simulink model "Redresseur_MLI_3Ph_MLI_antiwindup_relay"  (R2018b)
settings: Solver=ode8  StartTime=0.0  StopTime=0.3  FixedStep=1e-6  MaxStep=1e-6  RelTol=1e-3
undefined symbols (not defined in the file): C, Im, inverter_matrix, K, L, R, Ta, Td, Ti, V
libraries: simulink x1
settings Model: Creator=driss  LastModifiedBy=driss
settings SolverCC: ZeroCrossAlgorithm=Adaptive
settings DataIOCC: ReturnWorkspaceOutputs=on
settings DebuggingCC: MaxConsecutiveZCsMsg=none  UnconnectedInputMsg=none  UnconnectedOutputMsg=none  UnconnectedLineMsg=none
settings ModelReferenceCC: EnableRefExpFcnMdlSchedulingChecks=off
settings RTWCC: Description=Generic Real-Time Target

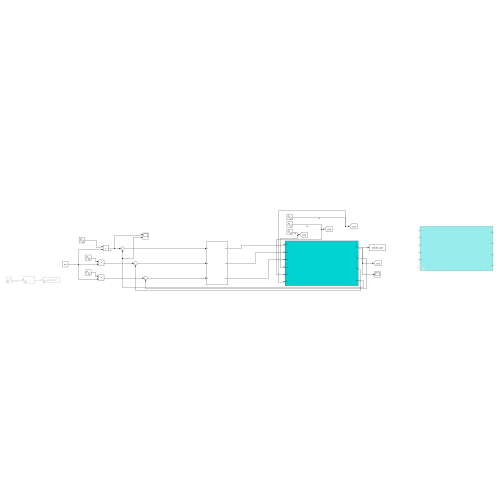
[thumbnail: Simulink's stored preview of the top-level diagram]
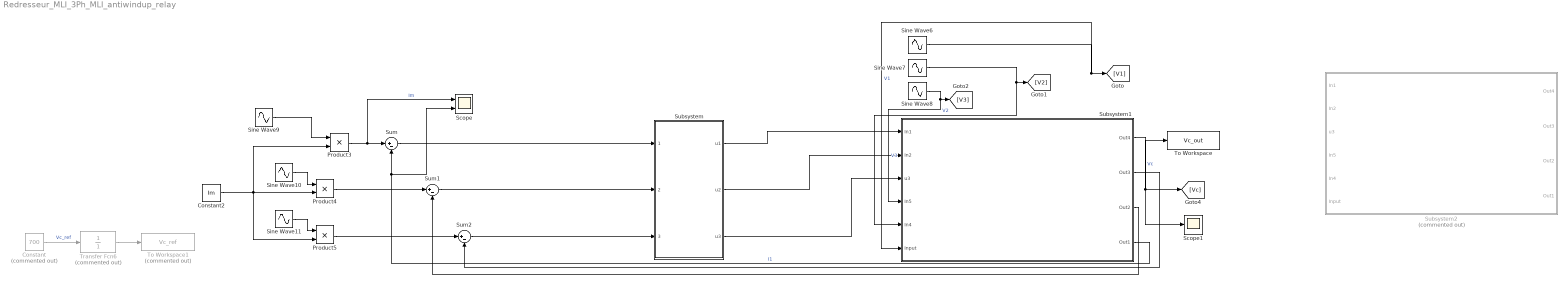
== system Redresseur_MLI_3Ph_MLI_antiwindup_relay ==
  Constant : Constant  Commented=on  Value=700
  Constant2 : Constant  Value=Im
  Product3 : Product
  Product4 : Product
  Product5 : Product
  Scope : Scope  NumInputPorts=2
  Scope1 : Scope
  Sine Wave10 : Sin  Frequency=2*50*pi  Phase=-2*pi/3  SampleTime=0
  Sine Wave11 : Sin  Frequency=2*50*pi  Phase=-4*pi/3  SampleTime=0
  Sine Wave6 : Sin  Amplitude=V*sqrt(2)  Frequency=2*50*pi  SampleTime=0
  Sine Wave7 : Sin  Amplitude=V*sqrt(2)  Frequency=2*50*pi  Phase=-2*pi/3  SampleTime=0
  Sine Wave8 : Sin  Amplitude=V*sqrt(2)  Frequency=2*50*pi  Phase=-4*pi/3  SampleTime=0
  Sine Wave9 : Sin  Frequency=2*50*pi  SampleTime=0
  Subsystem : Subsystem
  Subsystem1 : Subsystem
  Subsystem2 : Subsystem  Commented=on
  Sum : Sum  Inputs=|+-
  Sum1 : Sum  Inputs=|+-
  Sum2 : Sum  Inputs=|+-
  To Workspace : ToWorkspace  VariableName=Vc_out  SaveFormat=Timeseries  SampleTime=-1
  To Workspace1 : ToWorkspace  Commented=on  VariableName=Vc_ref  SaveFormat=Timeseries  SampleTime=-1
  Transfer Fcn6 : TransferFcn  Commented=on  Denominator=[0 1]
  wires:
  Constant/1 -> Transfer Fcn6/1  "Vc_ref"
  Sine Wave7/1 -> Subsystem1/5(In4), [V2]  "V2"
  Sine Wave8/1 -> Subsystem1/4(In5), [V3]  "V3"
  Sine Wave6/1 -> Subsystem1/6(Input), [V1]  "V1"
  Subsystem1/1(Out4) -> To Workspace/1, Scope1/1, [Vc]  "Vc"
  Sine Wave11/1 -> Product5/1
  Sine Wave10/1 -> Product4/1
  Sine Wave9/1 -> Product3/1
  Constant2/1 -> Product5/2, Product4/2, Product3/2
  Product3/1 -> Scope/1, Sum/1  "Im"
  Product4/1 -> Sum1/1
  Product5/1 -> Sum2/1
  Subsystem1/2(Out3) -> Sum2/2
  Subsystem1/3(Out2) -> Sum1/2
  Subsystem1/4(Out1) -> Scope/2, Sum/2  "I1"
  Transfer Fcn6/1 -> To Workspace1/1
  Subsystem/3(u3) -> Subsystem1/3(u3)
  Subsystem/2(u2) -> Subsystem1/2(In2)
  Subsystem/1(u1) -> Subsystem1/1(In1)
  Sum/1 -> Subsystem/1(1)
  Sum1/1 -> Subsystem/2(2)
  Sum2/1 -> Subsystem/3(3)

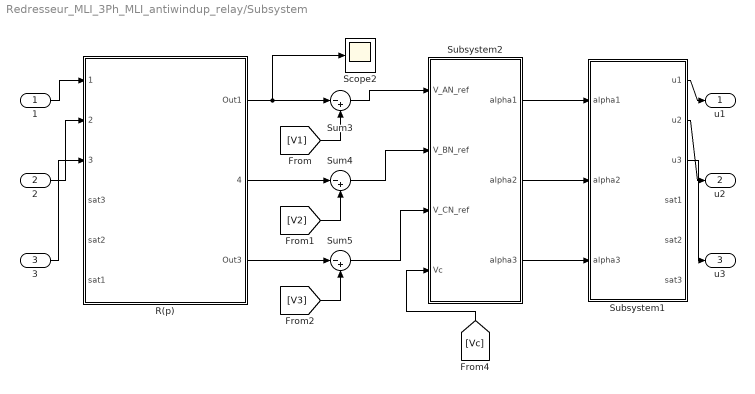
== system Redresseur_MLI_3Ph_MLI_antiwindup_relay/Subsystem ==
  1 : Inport
  2 : Inport  Port=2
  3 : Inport  Port=3
  R(p) : Subsystem
  Scope2 : Scope
  Subsystem1 : Subsystem
  Subsystem2 : Subsystem
  Sum3 : Sum  Inputs=|-+
  Sum4 : Sum  Inputs=|-+
  Sum5 : Sum  Inputs=|-+
  u1 : Outport
  u2 : Outport  Port=2
  u3 : Outport  Port=3
  wires:
  R(p)/2(4) -> Sum4/1
  R(p)/1(Out1) -> Scope2/1, Sum3/1
  Subsystem2/3(alpha3) -> Subsystem1/3(alpha3)
  [Vc] -> Subsystem2/4(Vc)
  Subsystem2/1(alpha1) -> Subsystem1/1(alpha1)
  R(p)/3(Out3) -> Sum5/1
  Subsystem2/2(alpha2) -> Subsystem1/2(alpha2)
  Subsystem1/1(u1) -> u1/1
  [V1] -> Sum3/2
  [V2] -> Sum4/2
  Sum3/1 -> Subsystem2/1(V_AN_ref)
  [V3] -> Sum5/2
  3/1 -> R(p)/3(3)
  Sum4/1 -> Subsystem2/2(V_BN_ref)
  Sum5/1 -> Subsystem2/3(V_CN_ref)
  Subsystem1/2(u2) -> u2/1
  Subsystem1/3(u3) -> u3/1
  2/1 -> R(p)/2(2)
  1/1 -> R(p)/1(1)

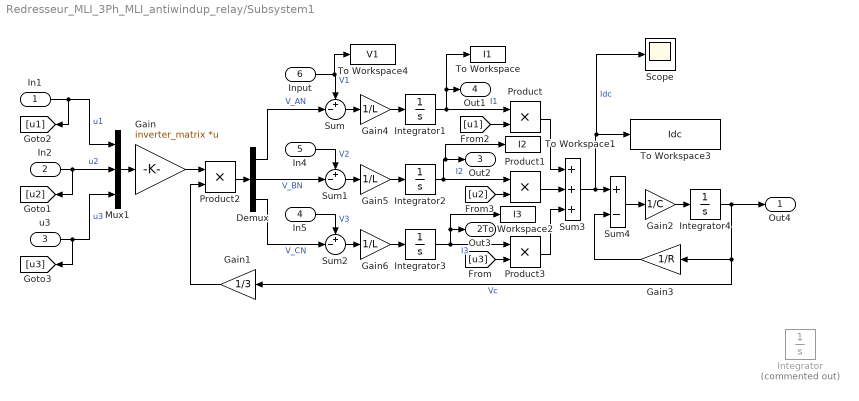
== system Redresseur_MLI_3Ph_MLI_antiwindup_relay/Subsystem1 ==
  In1 : Inport
  In2 : Inport  Port=2
  u3 : Inport  Port=3
  In5 : Inport  Port=4
  In4 : Inport  Port=5
  Input : Inport  Port=6
  Demux : Demux  Outputs=3
  Gain : Gain  Gain=inverter_matrix  Multiplication=Matrix(K*u)
  Gain1 : Gain  Gain=1/3
  Gain2 : Gain  Gain=1/C
  Gain3 : Gain  Gain=1/R
  Gain4 : Gain  Gain=1/L
  Gain5 : Gain  Gain=1/L
  Gain6 : Gain  Gain=1/L
  Integrator : Integrator  Commented=on  LimitOutput=on  LowerSaturationLimit=0
  Integrator1 : Integrator
  Integrator2 : Integrator
  Integrator3 : Integrator
  Integrator4 : Integrator  InitialCondition=V*sqrt(2)*sqrt(3)
  Mux1 : Mux  Inputs=3
  Product{,1..3} (4 alike) : Product
  Scope : Scope
  Sum : Sum  Inputs=+-|
  Sum1 : Sum  Inputs=+-|
  Sum2 : Sum  Inputs=+-|
  Sum3 : Sum  Inputs=+++
  Sum4 : Sum  Inputs=+-
  To Workspace : ToWorkspace  VariableName=I1  SaveFormat=Timeseries  SampleTime=-1
  To Workspace1 : ToWorkspace  VariableName=I2  SaveFormat=Timeseries  SampleTime=-1
  To Workspace2 : ToWorkspace  VariableName=I3  SaveFormat=Timeseries  SampleTime=-1
  To Workspace3 : ToWorkspace  VariableName=Idc  SaveFormat=Timeseries  SampleTime=-1
  To Workspace4 : ToWorkspace  VariableName=V1  SaveFormat=Timeseries  SampleTime=-1
  Out4 : Outport
  Out3 : Outport  Port=2
  Out2 : Outport  Port=3
  Out1 : Outport  Port=4
  wires:
  [u2] -> Product1/2
  [u1] -> Product/2
  Product2/1 -> Demux/1
  Gain6/1 -> Integrator3/1
  Gain5/1 -> Integrator2/1
  Gain4/1 -> Integrator1/1
  Gain3/1 -> Sum4/2
  Integrator4/1 -> Gain3/1, Gain1/1, Out4/1  "Vc"
  Gain2/1 -> Integrator4/1
  Sum4/1 -> Gain2/1
  Sum3/1 -> Sum4/1, Scope/1, To Workspace3/1  "Idc"
  Gain/1 -> Product2/1
  Gain1/1 -> Product2/2
  Product3/1 -> Sum3/3
  Product1/1 -> Sum3/2
  Product/1 -> Sum3/1
  [u3] -> Product3/2
  Mux1/1 -> Gain/1
  Integrator2/1 -> Out2/1, To Workspace1/1, Product1/1  "I2"
  Integrator3/1 -> Product3/1, Out3/1, To Workspace2/1  "I3"
  Integrator1/1 -> Product/1, Out1/1, To Workspace/1  "I1"
  Sum2/1 -> Gain6/1
  Sum1/1 -> Gain5/1
  Sum/1 -> Gain4/1
  In5/1 -> Sum2/1  "V3"
  In4/1 -> Sum1/1  "V2"
  Input/1 -> Sum/1, To Workspace4/1  "V1"
  Demux/1 -> Sum/2  "V_AN"
  Demux/3 -> Sum2/2  "V_CN"
  Demux/2 -> Sum1/2  "V_BN"
  In1/1 -> Mux1/1, [u1]  "u1"
  In2/1 -> Mux1/2, [u2]  "u2"
  u3/1 -> Mux1/3, [u3]  "u3"

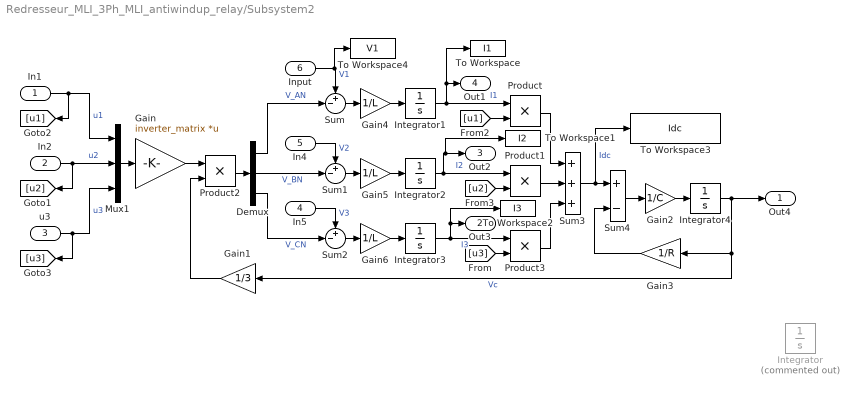
== system Redresseur_MLI_3Ph_MLI_antiwindup_relay/Subsystem2 ==
  In1 : Inport
  In2 : Inport  Port=2
  u3 : Inport  Port=3
  In5 : Inport  Port=4
  In4 : Inport  Port=5
  Input : Inport  Port=6
  Demux : Demux  Outputs=3
  Gain : Gain  Gain=inverter_matrix  Multiplication=Matrix(K*u)
  Gain1 : Gain  Gain=1/3
  Gain2 : Gain  Gain=1/C
  Gain3 : Gain  Gain=1/R
  Gain4 : Gain  Gain=1/L
  Gain5 : Gain  Gain=1/L
  Gain6 : Gain  Gain=1/L
  Integrator : Integrator  Commented=on  LimitOutput=on  LowerSaturationLimit=0
  Integrator1 : Integrator
  Integrator2 : Integrator
  Integrator3 : Integrator
  Integrator4 : Integrator  InitialCondition=V*sqrt(2)*sqrt(3)
  Mux1 : Mux  Inputs=3
  Product{,1..3} (4 alike) : Product
  Sum : Sum  Inputs=+-|
  Sum1 : Sum  Inputs=+-|
  Sum2 : Sum  Inputs=+-|
  Sum3 : Sum  Inputs=+++
  Sum4 : Sum  Inputs=+-
  To Workspace : ToWorkspace  VariableName=I1  SaveFormat=Timeseries  SampleTime=-1
  To Workspace1 : ToWorkspace  VariableName=I2  SaveFormat=Timeseries  SampleTime=-1
  To Workspace2 : ToWorkspace  VariableName=I3  SaveFormat=Timeseries  SampleTime=-1
  To Workspace3 : ToWorkspace  VariableName=Idc  SaveFormat=Timeseries  SampleTime=-1
  To Workspace4 : ToWorkspace  VariableName=V1  SaveFormat=Timeseries  SampleTime=-1
  Out4 : Outport
  Out3 : Outport  Port=2
  Out2 : Outport  Port=3
  Out1 : Outport  Port=4
  wires:
  u3/1 -> [u3], Mux1/3  "u3"
  In2/1 -> [u2], Mux1/2  "u2"
  In1/1 -> [u1], Mux1/1  "u1"
  Demux/2 -> Sum1/2  "V_BN"
  Demux/3 -> Sum2/2  "V_CN"
  Demux/1 -> Sum/2  "V_AN"
  Input/1 -> To Workspace4/1, Sum/1  "V1"
  In4/1 -> Sum1/1  "V2"
  In5/1 -> Sum2/1  "V3"
  Sum/1 -> Gain4/1
  Sum1/1 -> Gain5/1
  Sum2/1 -> Gain6/1
  Integrator1/1 -> To Workspace/1, Out1/1, Product/1  "I1"
  Integrator3/1 -> To Workspace2/1, Out3/1, Product3/1  "I3"
  Integrator2/1 -> Product1/1, To Workspace1/1, Out2/1  "I2"
  Mux1/1 -> Gain/1
  [u3] -> Product3/2
  Product/1 -> Sum3/1
  Product1/1 -> Sum3/2
  Product3/1 -> Sum3/3
  Gain1/1 -> Product2/2
  Gain/1 -> Product2/1
  Sum3/1 -> To Workspace3/1, Sum4/1  "Idc"
  Sum4/1 -> Gain2/1
  Gain2/1 -> Integrator4/1
  Integrator4/1 -> Out4/1, Gain1/1, Gain3/1  "Vc"
  Gain3/1 -> Sum4/2
  Gain4/1 -> Integrator1/1
  Gain5/1 -> Integrator2/1
  Gain6/1 -> Integrator3/1
  Product2/1 -> Demux/1
  [u1] -> Product/2
  [u2] -> Product1/2

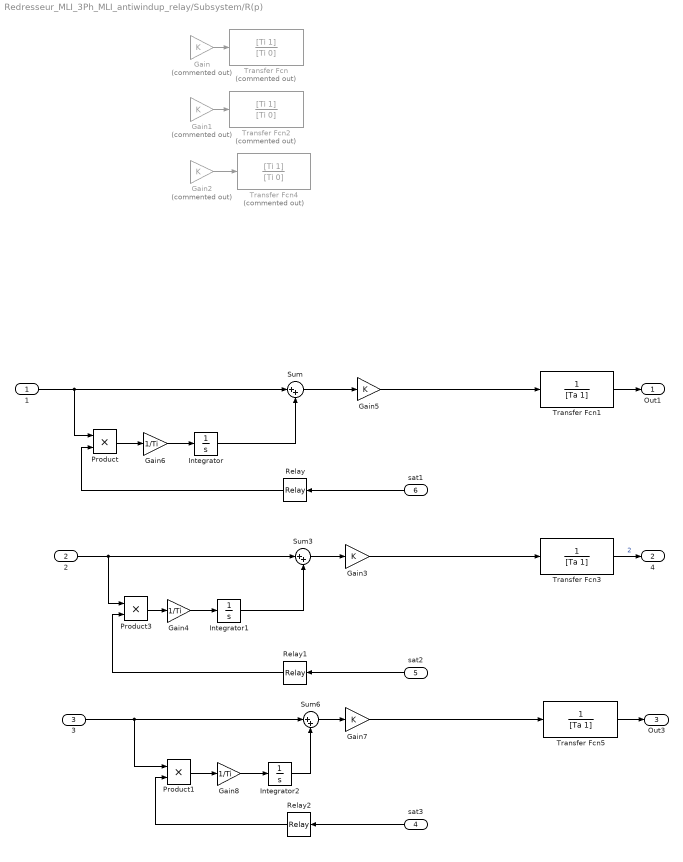
== system Redresseur_MLI_3Ph_MLI_antiwindup_relay/Subsystem/R(p) ==
  1 : Inport
  2 : Inport  Port=2
  3 : Inport  Port=3
  sat3 : Inport  Port=4
  sat2 : Inport  Port=5
  sat1 : Inport  Port=6
  Gain : Gain  Commented=on  Gain=K
  Gain1 : Gain  Commented=on  Gain=K
  Gain2 : Gain  Commented=on  Gain=K
  Gain3 : Gain  Gain=K
  Gain4 : Gain  Gain=1/Ti
  Gain5 : Gain  Gain=K
  Gain6 : Gain  Gain=1/Ti
  Gain7 : Gain  Gain=K
  Gain8 : Gain  Gain=1/Ti
  Integrator : Integrator  InitialCondition=1
  Integrator1 : Integrator  InitialCondition=1
  Integrator2 : Integrator
  Product : Product
  Product1 : Product
  Product3 : Product
  Relay : Relay  OnSwitchValue=1e-4  OffSwitchValue=-1e-4
  Relay1 : Relay  OnSwitchValue=1e-4  OffSwitchValue=-1e-4
  Relay2 : Relay  OnSwitchValue=1e-4  OffSwitchValue=-1e-4
  Sum : Sum  Inputs=|++
  Sum3 : Sum  Inputs=|++
  Sum6 : Sum  Inputs=|++
  Transfer Fcn : TransferFcn  Commented=on  Numerator=[Ti 1]  Denominator=[Ti 0]
  Transfer Fcn1 : TransferFcn  Denominator=[Ta 1]
  Transfer Fcn2 : TransferFcn  Commented=on  Numerator=[Ti 1]  Denominator=[Ti 0]
  Transfer Fcn3 : TransferFcn  Denominator=[Ta 1]
  Transfer Fcn4 : TransferFcn  Commented=on  Numerator=[Ti 1]  Denominator=[Ti 0]
  Transfer Fcn5 : TransferFcn  Denominator=[Ta 1]
  Out1 : Outport
  4 : Outport  Port=2
  Out3 : Outport  Port=3
  wires:
  Gain1/1 -> Transfer Fcn2/1
  Gain2/1 -> Transfer Fcn4/1
  Gain/1 -> Transfer Fcn/1
  Relay/1 -> Product/2
  Integrator2/1 -> Sum6/2
  Gain5/1 -> Transfer Fcn1/1
  Relay2/1 -> Product1/2
  Gain4/1 -> Integrator1/1
  sat2/1 -> Relay1/1
  Gain3/1 -> Transfer Fcn3/1
  Sum3/1 -> Gain3/1
  2/1 -> Product3/1, Sum3/1
  1/1 -> Product/1, Sum/1
  Sum6/1 -> Gain7/1
  Gain6/1 -> Integrator/1
  Gain8/1 -> Integrator2/1
  sat3/1 -> Relay2/1
  Product1/1 -> Gain8/1
  Integrator/1 -> Sum/2
  3/1 -> Product1/1, Sum6/1
  Gain7/1 -> Transfer Fcn5/1
  Integrator1/1 -> Sum3/2
  Transfer Fcn3/1 -> 4/1  "2"
  Transfer Fcn1/1 -> Out1/1
  Product3/1 -> Gain4/1
  Relay1/1 -> Product3/2
  sat1/1 -> Relay/1
  Transfer Fcn5/1 -> Out3/1
  Product/1 -> Gain6/1
  Sum/1 -> Gain5/1

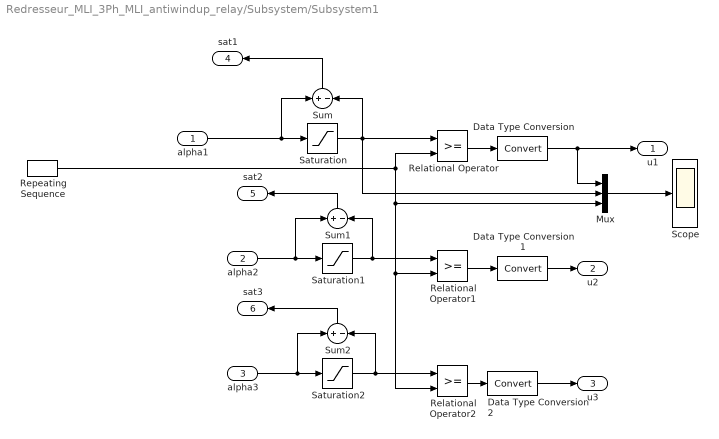
== system Redresseur_MLI_3Ph_MLI_antiwindup_relay/Subsystem/Subsystem1 ==
  alpha1 : Inport
  alpha2 : Inport  Port=2
  alpha3 : Inport  Port=3
  Data Type Conversion : DataTypeConversion
  Data Type Conversion1 : DataTypeConversion
  Data Type Conversion2 : DataTypeConversion
  Mux : Mux  Inputs=3
  Relational Operator : RelationalOperator  OutDataTypeStr=boolean  RndMeth=Simplest
  Relational Operator1 : RelationalOperator  OutDataTypeStr=boolean  RndMeth=Simplest
  Relational Operator2 : RelationalOperator  OutDataTypeStr=boolean  RndMeth=Simplest
  Repeating Sequence : simulink/Sources/Repeating Sequence  rep_seq_t=[0 Td/2 Td]  rep_seq_y=[1 0 1]
  Saturation : Saturate  UpperLimit=1  LowerLimit=0
  Saturation1 : Saturate  UpperLimit=1  LowerLimit=0
  Saturation2 : Saturate  UpperLimit=1  LowerLimit=0
  Scope : Scope
  Sum : Sum  Inputs=+-
  Sum1 : Sum  Inputs=+-
  Sum2 : Sum  Inputs=+-
  u1 : Outport
  u2 : Outport  Port=2
  u3 : Outport  Port=3
  sat1 : Outport  Port=4
  sat2 : Outport  Port=5
  sat3 : Outport  Port=6
  wires:
  Relational Operator/1 -> Data Type Conversion/1
  alpha1/1 -> Sum/1, Saturation/1
  Relational Operator1/1 -> Data Type Conversion1/1
  Relational Operator2/1 -> Data Type Conversion2/1
  Repeating Sequence/1 -> Relational Operator1/2, Relational Operator2/2, Mux/3, Relational Operator/2
  Saturation/1 -> Sum/2, Relational Operator/1, Mux/2
  Mux/1 -> Scope/1
  Data Type Conversion/1 -> Mux/1, u1/1
  Data Type Conversion1/1 -> u2/1
  Data Type Conversion2/1 -> u3/1
  Sum/1 -> sat1/1
  Sum1/1 -> sat2/1
  Saturation1/1 -> Sum1/2, Relational Operator1/1
  alpha2/1 -> Sum1/1, Saturation1/1
  alpha3/1 -> Sum2/1, Saturation2/1
  Saturation2/1 -> Sum2/2, Relational Operator2/1
  Sum2/1 -> sat3/1

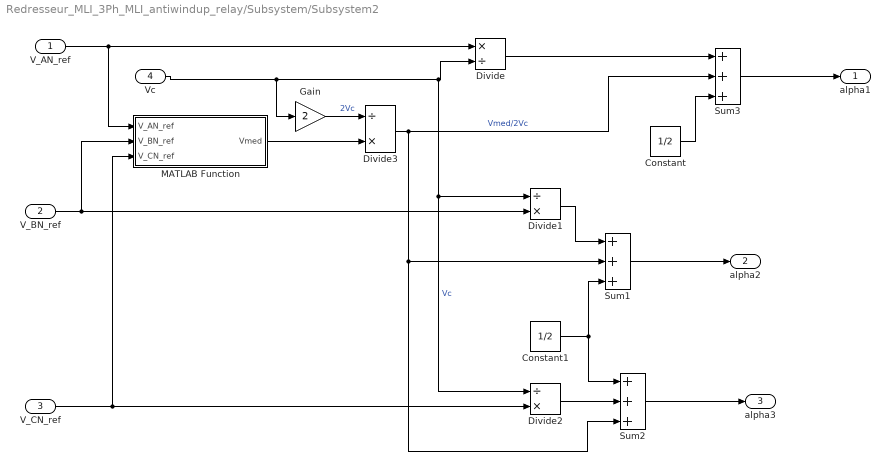
== system Redresseur_MLI_3Ph_MLI_antiwindup_relay/Subsystem/Subsystem2 ==
  V_AN_ref : Inport
  V_BN_ref : Inport  Port=2
  V_CN_ref : Inport  Port=3
  Vc : Inport  Port=4
  Constant : Constant  Value=1/2
  Constant1 : Constant  Value=1/2
  Divide : Product  Inputs=*/
  Divide1 : Product  Inputs=/*
  Divide2 : Product  Inputs=/*
  Divide3 : Product  Inputs=/*
  Gain : Gain  Gain=2
  MATLAB Function : MATLAB Function  TreatAsAtomicUnit=on
  Sum1 : Sum  Inputs=+++
  Sum2 : Sum  Inputs=+++
  Sum3 : Sum  Inputs=+++
  alpha1 : Outport
  alpha2 : Outport  Port=2
  alpha3 : Outport  Port=3
  wires:
  Sum3/1 -> alpha1/1
  V_AN_ref/1 -> MATLAB Function/1(V_AN_ref), Divide/1
  Divide/1 -> Sum3/1
  Constant/1 -> Sum3/3
  MATLAB Function/1(Vmed) -> Divide3/2
  Gain/1 -> Divide3/1  "2Vc"
  Constant1/1 -> Sum1/3, Sum2/1
  Sum1/1 -> alpha2/1
  Divide1/1 -> Sum1/1
  V_BN_ref/1 -> Divide1/2, MATLAB Function/2(V_BN_ref)
  Divide3/1 -> Sum2/3, Sum1/2, Sum3/2  "Vmed/2Vc"
  Vc/1 -> Divide2/1, Divide1/1, Divide/2, Gain/1  "Vc"
  V_CN_ref/1 -> MATLAB Function/3(V_CN_ref), Divide2/2
  Divide2/1 -> Sum2/2
  Sum2/1 -> alpha3/1

== matlab function Redresseur_MLI_3Ph_MLI_antiwindup_relay/Subsystem/Subsystem2/MATLAB Function ==
  data: V_AN_ref input; Vmed output; V_BN_ref input; V_CN_ref input
function Vmed = fcn(V_AN_ref,V_BN_ref,V_CN_ref)
     V_set = [V_AN_ref V_BN_ref V_CN_ref];
Vmed= -(min(V_set) + max(V_set));
